simulink model "tp394084"  (Simulink 3.0)
settings: Solver=ode1  StartTime=0.0  StopTime=inf  FixedStep=0.05  RelTol=1e-3  AbsTol=1e-6
libraries: udaq28LT_lib x1
settings Model: Creator=dmedonza  LastModifiedBy=mato  SaveFormat=Matrix  RTWTemplateMakefile=grt_vc.tmf  RTWOptions="-aEnforceIntegerDowncast=1 -aExtMode=0 -aExtModeTesting=0 -aFoldNonRolledExpr=1 -aForceParamTrailComments=0 -aGenerateComments=1 -aGenerateReport=0 -aIgnoreCustomStorageClasses=1 -aIncDataTypeInIds=0 -aIncHierarchyInIds=0 -aInlineInvariantSignals=0 -aInlinedPrmAccess=\"Literals\" -aLocalBlockOutputs=1 -aLogVarNameModifier=\"rt_\" -aMaxRTWIdLen=31 -aPrefixModelToSubsysFcnNames=1 -aRTWVerbose=1 -aRollThreshold=5 -aShowEliminatedStatements=0"

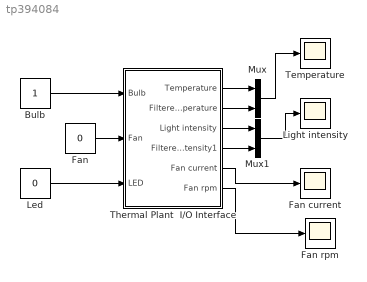
== system tp394084 ==
  Bulb : Constant  Value=1
  Fan : Constant  Value=0
  Fan current : Scope
      settings: TickLabels=on  TimeRange=auto  YMin=26  YMax=40  SaveName=y5  DataFormat=Matrix
  Fan rpm : Scope
      settings: TickLabels=on  TimeRange=auto  YMin=26  YMax=40  SaveName=y6  DataFormat=Matrix
  Led : Constant  Value=0
  Light intensity : Scope
      settings: TickLabels=on  TimeRange=auto  YMin=64  YMax=75  SaveName=y34  DataFormat=Matrix
  Mux : Mux  Inputs=2
  Mux1 : Mux  Inputs=2
  Temperature : Scope
      settings: TickLabels=on  TimeRange=10  YMin=27.65  YMax=28.65  SaveName=y12  DataFormat=Matrix
  Thermal Plant  I/O Interface : Subsystem
      mask Display: disp('Thermo-Optical\nPlant\nI/O Interface')
  wires:
  Mux/1 -> Temperature/1
  Mux1/1 -> Light intensity/1
  Bulb/1 -> Thermal Plant  I/O Interface/1(Bulb)
  Fan/1 -> Thermal Plant  I/O Interface/2(Fan)
  Led/1 -> Thermal Plant  I/O Interface/3(LED)
  Thermal Plant  I/O Interface/1(Temperature) -> Mux/1
  Thermal Plant  I/O Interface/2(Filtered  temperature) -> Mux/2
  Thermal Plant  I/O Interface/3(Light intensity) -> Mux1/1
  Thermal Plant  I/O Interface/4(Filtered  light intensity1) -> Mux1/2
  Thermal Plant  I/O Interface/5(Fan current) -> Fan current/1
  Thermal Plant  I/O Interface/6(Fan rpm) -> Fan rpm/1

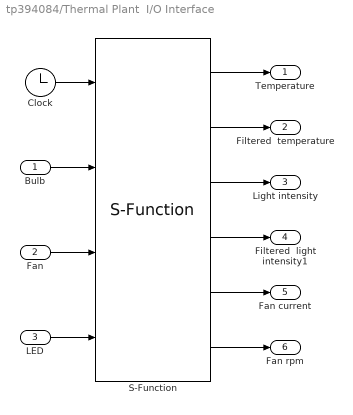
== system tp394084/Thermal Plant  I/O Interface ==
  Bulb : Inport  Port=1  PortWidth=-1  SampleTime=-1  DataType=auto
      settings: SignalType=auto
  Fan : Inport  Port=2  PortWidth=-1  SampleTime=-1  DataType=auto
      settings: SignalType=auto
  LED : Inport  Port=3  PortWidth=-1  SampleTime=-1  DataType=auto
      settings: SignalType=auto
  Clock : Clock
      settings: DisplayTime=off  Decimation=10
  S-Function : udaq28LT_lib/S-Function  Priority=1  com_port=COM4  Ts=0.05  events_ot=2  rd_timeout=25  matlab_prior=ABOVE_NORMAL_PRIORITY  warning=on  printout=off
  Temperature : Outport  Port=1
  Filtered  temperature : Outport  Port=2
  Light intensity : Outport  Port=3
  Filtered  light intensity1 : Outport  Port=4
  Fan current : Outport  Port=5
  Fan rpm : Outport  Port=6
  wires:
  S-Function/1 -> Temperature/1
  S-Function/2 -> Filtered  temperature/1
  Clock/1 -> S-Function/1
  Bulb/1 -> S-Function/2
  Fan/1 -> S-Function/3
  S-Function/3 -> Light intensity/1
  S-Function/4 -> Filtered  light intensity1/1
  S-Function/5 -> Fan current/1
  S-Function/6 -> Fan rpm/1
  LED/1 -> S-Function/4
